simulink model "ex5"  (R2020a)
settings: Solver=VariableStepAuto  StartTime=0.0  StopTime=100  RelTol=1e-3
values from neighbouring files (symbols this model uses):
  c = 0    [ex 5 residual solution.m]
  k = 100    [ex 5 residual solution.m]
  m = 2    [ex 5 residual solution.m]
libraries: simulink x2, simulink_extras x2
settings Model: Creator=EREN  LastModifiedBy=EREN

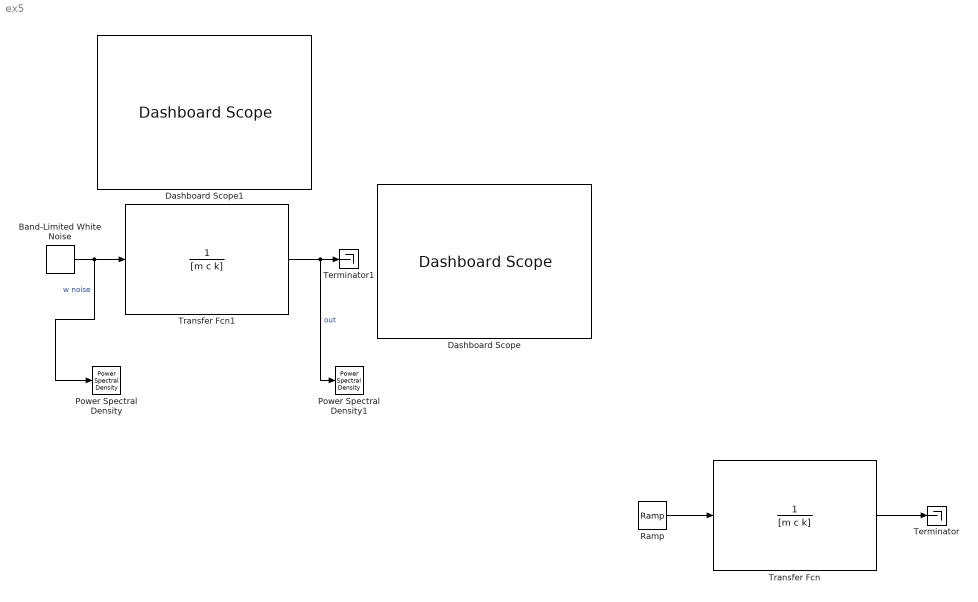
== system ex5 ==
  Band-Limited White Noise : simulink/Sources/Band-Limited White Noise  Cov=[0.1]  Ts=0.01  seed=[23341]
  Dashboard Scope : DashboardScope
  Dashboard Scope1 : DashboardScope
  Power Spectral Density : simulink_extras/Additional Sinks/Power Spectral Density  npts=128  fftpts=512  HowOften=64  sampleT=0.1
      settings: SourceProductBaseCode=SL
  Power Spectral Density1 : simulink_extras/Additional Sinks/Power Spectral Density  npts=128  fftpts=512  HowOften=64  sampleT=0.1
      settings: SourceProductBaseCode=SL
  Ramp : simulink/Sources/Ramp  slope=10  start=0  InitialOutput=0
  Terminator : Terminator
  Terminator1 : Terminator
  Transfer Fcn : TransferFcn  Denominator=[m c k]
  Transfer Fcn1 : TransferFcn  Denominator=[m c k]
  wires:
  Ramp/1 -> Transfer Fcn/1
  Transfer Fcn/1 -> Terminator/1
  Transfer Fcn1/1 -> Power Spectral Density1/1, Terminator1/1  "out"
  Band-Limited White Noise/1 -> Power Spectral Density/1, Transfer Fcn1/1  "w noise"
